simulink model "Actuators"  (R2023a)
settings: Solver=VariableStepAuto  StartTime=0.0  StopTime=10.0  RelTol=1e-3
settings Model: Creator=aan18022  LastModifiedBy=aan18022

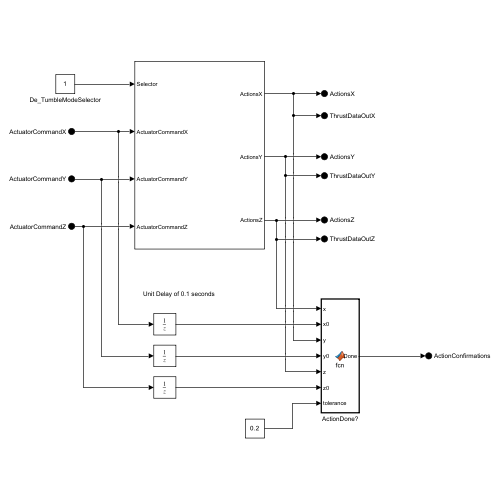
[thumbnail: Simulink's stored preview of the top-level diagram]
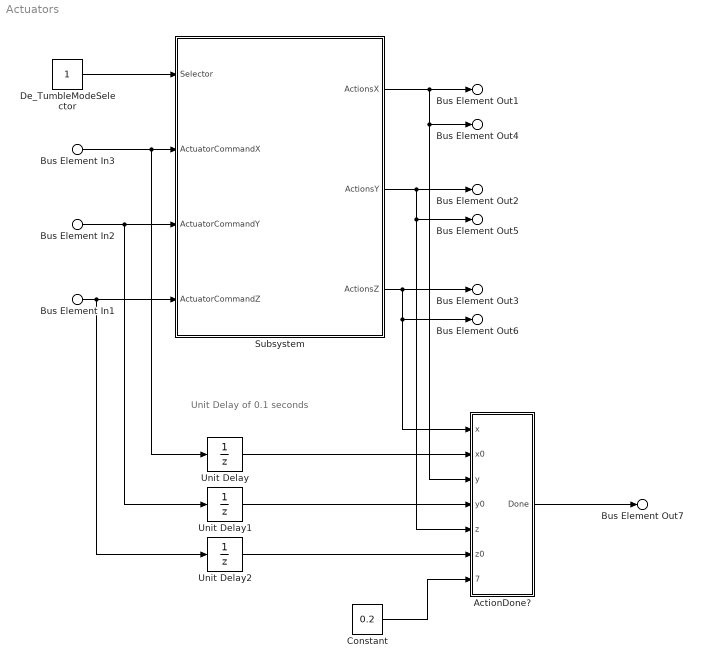
== system Actuators ==
  note: Unit Delay of 0.1 seconds
  Bus Element In3 : Inport  PortName=ActuatorCommandX
  Bus Element In2 : Inport  Port=2  PortName=ActuatorCommandY
  Bus Element In1 : Inport  Port=3  PortName=ActuatorCommandZ
  ActionDone? : MATLAB Function  TreatAsAtomicUnit=on
  Constant : Constant  Value=0.2
  De_TumbleModeSelector : Constant
  Subsystem : Subsystem
  Unit Delay : UnitDelay  SampleTime=0.1  HasFrameUpgradeWarning=on
  Unit Delay1 : UnitDelay  SampleTime=0.1  HasFrameUpgradeWarning=on
  Unit Delay2 : UnitDelay  SampleTime=0.1  HasFrameUpgradeWarning=on
  Bus Element Out1 : Outport  PortName=ActionsX
  Bus Element Out2 : Outport  Port=2  PortName=ActionsY
  Bus Element Out3 : Outport  Port=3  PortName=ActionsZ
  Bus Element Out4 : Outport  Port=4  PortName=ThrustDataOutX
  Bus Element Out5 : Outport  Port=5  PortName=ThrustDataOutY
  Bus Element Out6 : Outport  Port=6  PortName=ThrustDataOutZ
  Bus Element Out7 : Outport  Port=7  PortName=ActionConfirmations
  wires:
  Subsystem/1(ActionsX) -> Bus Element Out1/1, ActionDone?/3(y), Bus Element Out4/1
  Subsystem/3(ActionsZ) -> Bus Element Out3/1, Bus Element Out6/1, ActionDone?/1(x)
  Subsystem/2(ActionsY) -> Bus Element Out2/1, ActionDone?/5(z), Bus Element Out5/1
  Bus Element In3/1 -> Unit Delay/1, Subsystem/2(ActuatorCommandX)
  Bus Element In2/1 -> Unit Delay1/1, Subsystem/3(ActuatorCommandY)
  Bus Element In1/1 -> Unit Delay2/1, Subsystem/4(ActuatorCommandZ)
  De_TumbleModeSelector/1 -> Subsystem/1(Selector)
  Unit Delay/1 -> ActionDone?/2(x0)
  Unit Delay1/1 -> ActionDone?/4(y0)
  Unit Delay2/1 -> ActionDone?/6(z0)
  Constant/1 -> ActionDone?/7(tolerance)
  ActionDone?/1(Done) -> Bus Element Out7/1

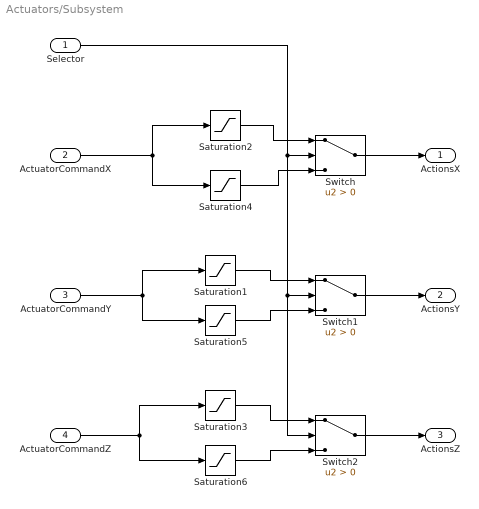
== system Actuators/Subsystem ==
  Selector : Inport
  ActuatorCommandX : Inport  Port=2
  ActuatorCommandY : Inport  Port=3
  ActuatorCommandZ : Inport  Port=4
  Saturation1 : Saturate  UpperLimit=1  LowerLimit=-1
  Saturation2 : Saturate  UpperLimit=1  LowerLimit=-1
  Saturation3 : Saturate  UpperLimit=1  LowerLimit=-1
  Saturation4 : Saturate  UpperLimit=0.25  LowerLimit=-0.25
  Saturation5 : Saturate  UpperLimit=0.25  LowerLimit=-0.25
  Saturation6 : Saturate  UpperLimit=0.25  LowerLimit=-0.25
  Switch : Switch  Criteria=u2 > Threshold  SaturateOnIntegerOverflow=off  InputSameDT=off
  Switch1 : Switch  Criteria=u2 > Threshold  SaturateOnIntegerOverflow=off  InputSameDT=off
  Switch2 : Switch  Criteria=u2 > Threshold  SaturateOnIntegerOverflow=off  InputSameDT=off
  ActionsX : Outport
  ActionsY : Outport  Port=2
  ActionsZ : Outport  Port=3
  wires:
  ActuatorCommandX/1 -> Saturation2/1, Saturation4/1
  ActuatorCommandY/1 -> Saturation5/1, Saturation1/1
  ActuatorCommandZ/1 -> Saturation6/1, Saturation3/1
  Saturation2/1 -> Switch/1
  Saturation4/1 -> Switch/3
  Selector/1 -> Switch/2, Switch1/2, Switch2/2
  Switch/1 -> ActionsX/1
  Saturation1/1 -> Switch1/1
  Saturation5/1 -> Switch1/3
  Saturation3/1 -> Switch2/1
  Saturation6/1 -> Switch2/3
  Switch2/1 -> ActionsZ/1
  Switch1/1 -> ActionsY/1

== matlab function Actuators/ActionDone? ==
  data: x input; x0 input; y input; y0 input; Done output; z input; z0 input; tolerance input
function Done = fcn(x,x0,y,y0,z,z0,tolerance)

upperX = x0 + tolerance;
lowX = x0 - tolerance;
upperY = y0 + tolerance;
lowY = y0 - tolerance;
upperZ = z0 + tolerance;
lowZ = z0 - tolerance;

if (x <= upperX && x >= lowX)
    xTerm = 1;
else
    xTerm = 0;
end

if (y <= upperY && y >= lowY)
    yTerm = 1;
else
    yTerm = 0;
end

if (z <= upperZ && z >= lowZ)
    zTerm = 1;
else
    zTerm = 0;
end

Done = xTerm * yTerm * zTerm; %% Will remain 0 until all terms are 1 which means that the old value is the same as the present value and the command is stabilised.
